simulink model "scp_comm"  (R2025b)
settings: Solver=ode4  StartTime=0.0  StopTime=50  FixedStep=scp_h  RelTol=1e-3
values from neighbouring files (symbols this model uses):
  scp_h = 0.01    [build_scp_comm.m]
  scp_seed = 2026    [build_scp_comm.m]
  scp_threshold = 0.6    [build_scp_comm.m]
settings Model: Creator=yuexi  LastModifiedBy=yuexi

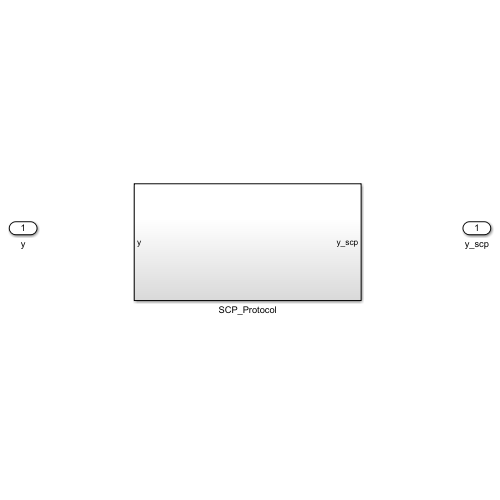
[thumbnail: Simulink's stored preview of the top-level diagram]
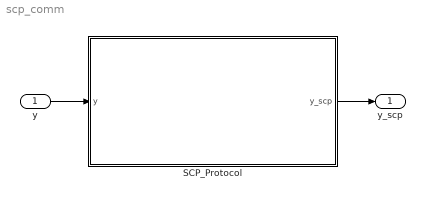
== system scp_comm ==
  y : Inport
  SCP_Protocol : Subsystem
  y_scp : Outport
  wires:
  y/1 -> SCP_Protocol/1(y)
  SCP_Protocol/1(y_scp) -> y_scp/1

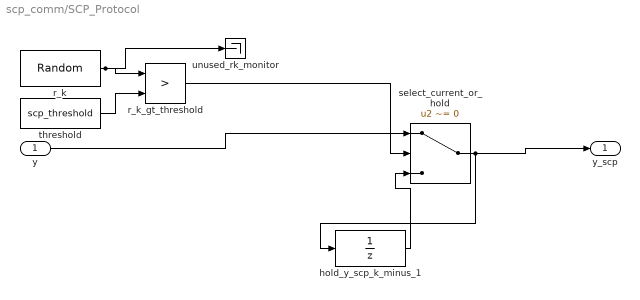
== system scp_comm/SCP_Protocol ==
  y : Inport
  hold_y_scp_k_minus_1 : UnitDelay  SampleTime=scp_h  HasFrameUpgradeWarning=on
  r_k : UniformRandomNumber  Minimum=0  Seed=scp_seed  SampleTime=scp_h
  r_k_gt_threshold : RelationalOperator  Operator=>  OutDataTypeStr=boolean  RndMeth=Simplest  InputSameDT=off
  select_current_or_hold : Switch  Criteria=u2 ~= 0  Threshold=0.5  SaturateOnIntegerOverflow=off  InputSameDT=off
  threshold : Constant  Value=scp_threshold
  unused_rk_monitor : Terminator
  y_scp : Outport
  wires:
  r_k/1 -> r_k_gt_threshold/1, unused_rk_monitor/1
  threshold/1 -> r_k_gt_threshold/2
  y/1 -> select_current_or_hold/1
  r_k_gt_threshold/1 -> select_current_or_hold/2
  hold_y_scp_k_minus_1/1 -> select_current_or_hold/3
  select_current_or_hold/1 -> y_scp/1, hold_y_scp_k_minus_1/1
